simulink model "dspsdadc3"  (Simulink 7.4)
settings: Solver=ode45  SolverMode=SingleTasking  StartTime=0.0  StopTime=.1  FixedStep=1/512000  RelTol=1e-4
libraries: dspmlti4 x3, simulink x2, dspobslib x1, dspsnks4 x1
settings Model: Creator=don  LastModifiedBy=Dick  ExtModeTrigMode=oneshot  ExtModeArmWhenConnect=off
settings SolverCC: InitialStep=1e-8
settings DataIOCC: LimitDataPoints=off  SaveOutput=off  SaveTime=off  SignalLoggingName=sigsOut
settings OptimizationCC: BlockReduction=off  BooleanDataType=off  InlineInvariantSignals=on  InitFltsAndDblsToZero=on
settings DebuggingCC: SaveWithParameterizedLinksMsg=none  SignalResolutionControl=TryResolveAllWithWarning  SolverPrmCheckMsg=none  MultiTaskDSMMsg=warning  MultiTaskCondExecSysMsg=none  IntegerOverflowMsg=none  StrictBusMsg=None
settings HardwareCC: TargetUnknown=on
settings RTWCC: IncludeERTFirstTime=on
settings GRTTargetCC: TargetFcnLib=ansi_tfl_tmw.mat

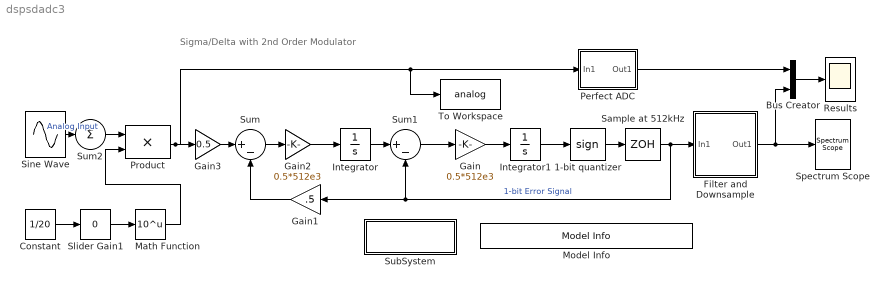
== system dspsdadc3 ==
  note: Sigma/Delta with 2nd Order Modulator
  1-bit quantizer : Signum
  Bus Creator : BusCreator  Inputs=2
  Constant : Constant  Value=1/20  OutDataType=sfix(16)  OutScaling=2^0
  Filter and Downsample : Subsystem
  Gain : Gain  Gain=0.5*512e3  ParameterDataType=sfix(16)  ParameterScaling=2^0  OutDataType=sfix(16)  OutScaling=2^0  SaturateOnIntegerOverflow=on  OutDataTypeStr=Inherit: Same as input  ParamDataTypeStr=Inherit: Same as input
  Gain1 : Gain  Gain=.5  ParameterDataType=sfix(16)  ParameterScaling=2^0  OutDataType=sfix(16)  OutScaling=2^0  SaturateOnIntegerOverflow=on  OutDataTypeStr=Inherit: Same as input  ParamDataTypeStr=Inherit: Same as input
  Gain2 : Gain  Gain=0.5*512e3  ParameterDataType=sfix(16)  ParameterScaling=2^0  OutDataType=sfix(16)  OutScaling=2^0  SaturateOnIntegerOverflow=on  OutDataTypeStr=Inherit: Same as input  ParamDataTypeStr=Inherit: Same as input
  Gain3 : Gain  Gain=0.5  ParameterDataType=sfix(16)  ParameterScaling=2^0  OutDataType=sfix(16)  OutScaling=2^0  SaturateOnIntegerOverflow=on  OutDataTypeStr=Inherit: Same as input  ParamDataTypeStr=Inherit: Same as input
  Integrator : Integrator
  Integrator1 : Integrator
  Math Function : Math  Operator=10^u  OutDataType=sfix(16)  OutScaling=2^0  SaturateOnIntegerOverflow=on
  Model Info : simulink/Model-Wide Utilities/Model Info  SystemSampleTime=-1  InitialBlockCM=none  BlockCM=none  Frame=on  DisplayStringWithTags=Copywrite 2005-2010 The MathWorks, Inc.  HorizontalTextAlignment=Center  LeftAlignmentValue=0.5  SourceBlockDiagram=dspsdadc3  TagMaxNumber=20
  Perfect ADC : Subsystem
  Product : Product  OutDataType=sfix(16)  OutScaling=2^0  SaturateOnIntegerOverflow=on  OutDataTypeStr=Inherit: Same as first input
  Results : Scope
      settings: TimeRange=0.015  YMin=-1  YMax=1  DataFormat=Array
  Sample at 512kHz : ZeroOrderHold  SampleTime=1/512000
  Sine Wave : Sin  Amplitude=[1 1]*0.5  Bias=0  Frequency=[1500 1750]*2*pi  Phase=0  Samples=10  SampleTime=0  Offset=0
  Slider Gain1 : simulink/Math Operations/Slider Gain  SystemSampleTime=-1  low=-100  gain=0  high=10
  Spectrum Scope : dspsnks4/Spectrum Scope  DialogController=dspdialog.SpectrumScope  DialogControllerArgs=DataTag3  SystemSampleTime=-1  ScopeProperties=off  Domain=Frequency  HorizSpan=1  UseBuffer=on  BufferSize=512  Overlap=0  inpFftLenInherit=off  FFTlength=128  numAvg=1  DisplayProperties=off  AxisGrid=on  Memory=off  FrameNumber=on  AxisLegend=off  AxisZoom=off  OpenScopeAtSimStart=on  OpenScopeImmediately=off  FigPos=[14 34 560 276]  AxisProperties=on  XUnits=Hertz  XRange=[0...Fs/2]  XDisplay=0  InheritXIncr=on  XIncr=1.0  XLabel=Samples  XLimit=Auto  YUnits=dB  XMax=1  XMin=0  YLabel=Magnitude, dB  LineProperties=off  LineColors=[1 0 1]|[1 0 0]  wintypeSpecScope=Hann  RsSpecScope=50  betaSpecScope=5  winsampSpecScope=Periodic  XAxisParamsVer=6.8
      settings: YMin=-80  YMax=20
  SubSystem : Subsystem
      settings: OpenFcn=plot_signal
      mask Display: disp('plot signal')
  Sum : Sum  Inputs=|+-  OutDataType=sfix(16)  OutScaling=2^0  SaturateOnIntegerOverflow=on  InputSameDT=on  OutDataTypeStr=Inherit: Same as first input
  Sum1 : Sum  Inputs=|+-  OutDataType=sfix(16)  OutScaling=2^0  SaturateOnIntegerOverflow=on  InputSameDT=on  OutDataTypeStr=Inherit: Same as first input
  Sum2 : Sum  Inputs=1  OutDataType=sfix(16)  OutScaling=2^0  SaturateOnIntegerOverflow=on  InputSameDT=on  OutDataTypeStr=Inherit: Same as first input
  To Workspace : ToWorkspace  VariableName=analog  SampleTime=-1  SaveFormat=Structure With Time
  wires:
  Filter and Downsample/1(Out1) -> Bus Creator/2, Spectrum Scope/1
  Sine Wave/1 -> Sum2/1  "Analog Input"
  1-bit quantizer/1 -> Sample at 512kHz/1
  Sample at 512kHz/1 -> Filter and Downsample/1(In1), Sum1/2, Gain1/1  "1-bit Error Signal"
  Sum/1 -> Gain2/1
  Bus Creator/1 -> Results/1
  Perfect ADC/1(Out1) -> Bus Creator/1
  Integrator1/1 -> 1-bit quantizer/1
  Integrator/1 -> Sum1/1
  Sum1/1 -> Gain/1
  Gain/1 -> Integrator1/1
  Gain1/1 -> Sum/2
  Gain2/1 -> Integrator/1
  Gain3/1 -> Sum/1
  Product/1 -> Gain3/1, Perfect ADC/1(In1), To Workspace/1
  Sum2/1 -> Product/1
  Constant/1 -> Slider Gain1/1
  Slider Gain1/1 -> Math Function/1
  Math Function/1 -> Product/2

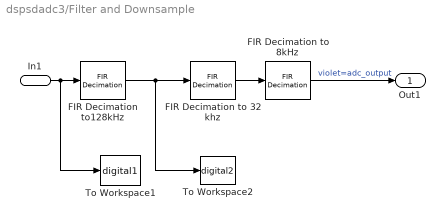
== system dspsdadc3/Filter and Downsample ==
  In1 : Inport  OutDataType=sfix(16)  OutScaling=2^0
  FIR Decimation to 32 khz : dspmlti4/FIR Decimation  DialogController=dspdialog.FIRDecimation  DialogControllerArgs=DataTag0  h=fir1(31, 0.15)  D=4  filtStruct=Direct form  framing=Maintain input frame size  outputBufInitCond=0  roundingMode=Floor  overflowMode=off  FilterSource=Specify via dialog  FilterObject=Hm_firdecim
  FIR Decimation to 8kHz : dspmlti4/FIR Decimation  DialogController=dspdialog.FIRDecimation  DialogControllerArgs=DataTag1  h=fir1(31, 0.15)  D=4  filtStruct=Direct form  framing=Maintain input frame size  outputBufInitCond=0  roundingMode=Floor  overflowMode=off  FilterSource=Specify via dialog  FilterObject=Hm_firdecim
  FIR Decimation to128kHz : dspmlti4/FIR Decimation  DialogController=dspdialog.FIRDecimation  DialogControllerArgs=DataTag2  h=fir1(31, 0.15)  D=4  filtStruct=Direct form  framing=Maintain input frame size  outputBufInitCond=0  roundingMode=Floor  overflowMode=off  FilterSource=Specify via dialog  FilterObject=Hm_firdecim
  To Workspace1 : ToWorkspace  VariableName=digital1  SampleTime=-1  SaveFormat=Structure With Time
  To Workspace2 : ToWorkspace  VariableName=digital2  SampleTime=-1  SaveFormat=Structure With Time
  Out1 : Outport  OutDataType=sfix(16)  OutScaling=2^0
  wires:
  FIR Decimation to 32 khz/1 -> FIR Decimation to 8kHz/1
  FIR Decimation to128kHz/1 -> FIR Decimation to 32 khz/1, To Workspace2/1
  In1/1 -> FIR Decimation to128kHz/1, To Workspace1/1
  FIR Decimation to 8kHz/1 -> Out1/1  "violet=adc_output"

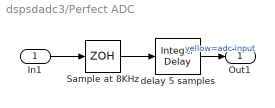
== system dspsdadc3/Perfect ADC ==
  In1 : Inport  OutDataType=sfix(16)  OutScaling=2^0
  Sample at 8KHz : ZeroOrderHold  SampleTime=1/8000
  delay 5 samples : dspobslib/Integer Delay  delay=5  ic=0  reset_popup=None
  Out1 : Outport  OutDataType=sfix(16)  OutScaling=2^0
  wires:
  Sample at 8KHz/1 -> delay 5 samples/1
  In1/1 -> Sample at 8KHz/1
  delay 5 samples/1 -> Out1/1  "yellow=adc input"

== system dspsdadc3/SubSystem ==
